simulink model "EZS4_template"  (R2017b)
settings: Solver=ode3  StartTime=0.0  StopTime=inf  RelTol=1e-3  EnableMultiTasking=on
libraries: arduinolib x13
settings Model: ExtModeTrigDuration=2  Creator=hartmann  LastModifiedBy=tanja
settings DataIOCC: LimitDataPoints=on  SaveFormat=Array
settings OptimizationCC: PassReuseOutputArgsThreshold=0  ExpressionDepthLimit=2147483647  MaxStackSize=64
settings DebuggingCC: UnderspecifiedInitializationDetection=Classic  MergeDetectMultiDrivingBlocksExec=none  ParameterTunabilityLossMsg=error  StateNameClashWarn=warning  SFUnexpectedBacktrackingDiag=warning  SFNoUnconditionalDefaultTransitionDiag=warning  SFExecutionAtInitializationDiag=none
settings HardwareCC: ProdBitPerInt=16  ProdBitPerPointer=16  ProdBitPerSizeT=16  ProdBitPerPtrDiffT=16  ProdLargestAtomicFloat=None  ProdWordSize=8  ProdHWDeviceType=Atmel->AVR  UseEmbeddedCoderFeatures=off  UseSimulinkCoderFeatures=off
settings ModelReferenceCC: PropagateSignalLabelsOutOfModel=off
settings SFSimCC: MATLABDynamicMemAlloc=off
settings RTWCC: SystemTargetFile=ert.tlc  HardwareBoard=Arduino Mega 2560  TLCOptions=-aInlineSetEventsForThisBaseRateFcn=TLC_FALSE -aSuppressMultiTaskScheduler=TLC_FALSE -aRateBasedStepFcn=1  TemplateMakefile=ert_default_tmf  GenerateReport=on  RTWVerbose=off  Toolchain=Arduino AVR  BuildConfiguration=Faster Runs  LaunchReport=on
settings CodeAppCC: ForceParamTrailComments=on  OperatorAnnotations=on
settings ERTTargetCC: ERTCustomFileBanners=off  SupportContinuousTime=on  SupportNonInlinedSFcns=on  RemoveResetFunc=off  SupportVariableSizeSignals=on  ModelStepFunctionPrototypeControlCompliant=off
settings ConfigComp: CovMetricSettings=dw  CovHtmlReporting=on  CovSaveCumulativeToWorkspaceVar=on  CovSaveSingleToWorkspaceVar=on  CovExternalEMLEnable=off  CovSFcnEnable=off

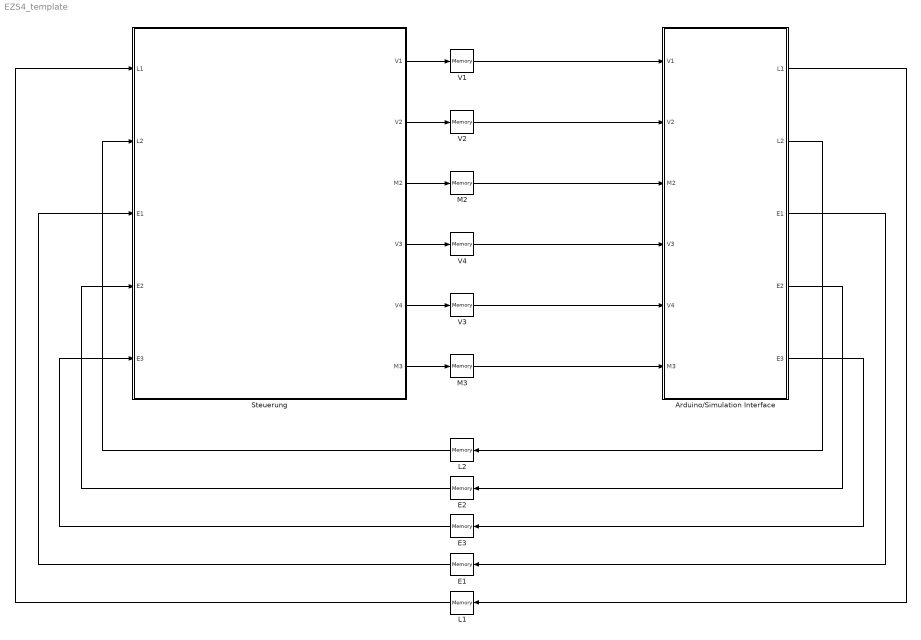
== system EZS4_template ==
  Arduino/Simulation Interface : Subsystem
  E1 : Memory
  E2 : Memory
  E3 : Memory
  L1 : Memory
  L2 : Memory
  M2 : Memory
  M3 : Memory
  Steuerung : Stateflow chart  TreatAsAtomicUnit=on
  V{1..4} (4 alike) : Memory
  wires:
  Steuerung/1(V1) -> V1/1
  Steuerung/2(V2) -> V2/1
  Steuerung/3(M2) -> M2/1
  Steuerung/6(M3) -> M3/1
  L1/1 -> Steuerung/1(L1)
  E1/1 -> Steuerung/3(E1)
  E3/1 -> Steuerung/5(E3)
  E2/1 -> Steuerung/4(E2)
  L2/1 -> Steuerung/2(L2)
  M3/1 -> Arduino/Simulation Interface/6("M3 ")
  V3/1 -> Arduino/Simulation Interface/5(V4)
  V4/1 -> Arduino/Simulation Interface/4(V3)
  M2/1 -> Arduino/Simulation Interface/3(M2)
  V2/1 -> Arduino/Simulation Interface/2(V2)
  V1/1 -> Arduino/Simulation Interface/1(V1)
  Arduino/Simulation Interface/1(L1) -> L1/1
  Arduino/Simulation Interface/2(L2) -> L2/1
  Arduino/Simulation Interface/3(E1) -> E1/1
  Arduino/Simulation Interface/4(E2) -> E2/1
  Arduino/Simulation Interface/5(E3) -> E3/1
  Steuerung/5(V4) -> V3/1
  Steuerung/4(V3) -> V4/1

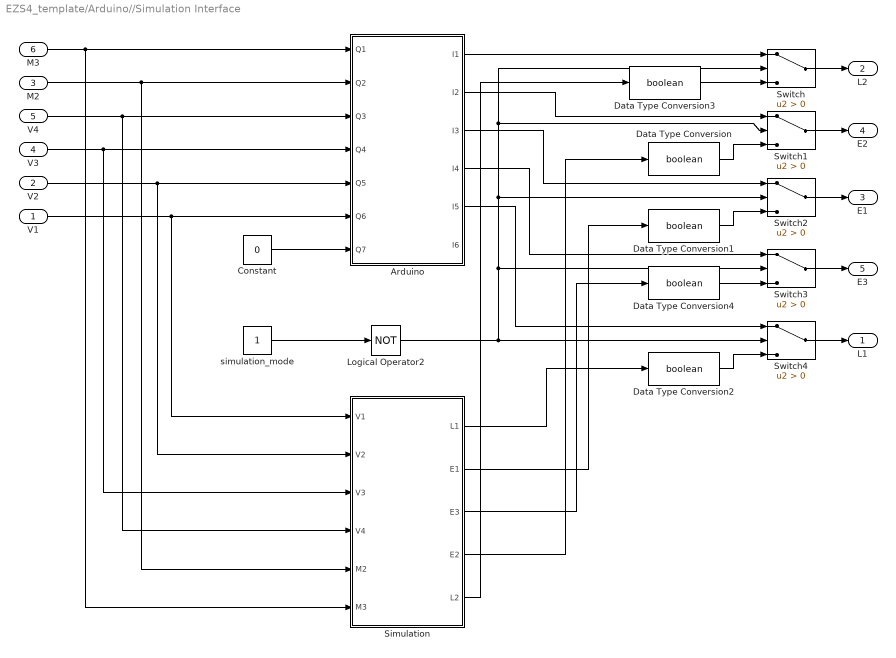
== system EZS4_template/Arduino//Simulation Interface ==
  V1 : Inport
  V2 : Inport  Port=2
  M2 : Inport  Port=3
  V3 : Inport  Port=4
  V4 : Inport  Port=5
  "M3 " : Inport  Port=6
  Arduino : Subsystem
  Constant : Constant  Value=0
  Data Type Conversion{,1..4} (5 alike) : DataTypeConversion  OutDataTypeStr=boolean
  Logical Operator2 : Logic  Operator=NOT  AllPortsSameDT=off  OutDataTypeStr=boolean
  Simulation : Stateflow chart  TreatAsAtomicUnit=on
  Switch{,1..4} (5 alike) : Switch  Criteria=u2 > Threshold
  simulation_mode : Constant
  L1 : Outport
  L2 : Outport  Port=2
  E1 : Outport  Port=3
  E2 : Outport  Port=4
  E3 : Outport  Port=5
  wires:
  Simulation/5(L2) -> Data Type Conversion3/1
  Switch/1 -> L2/1
  simulation_mode/1 -> Logical Operator2/1
  Arduino/1(I1) -> Switch/1
  Simulation/4(E2) -> Data Type Conversion/1
  Switch1/1 -> E2/1
  Arduino/2(I2) -> Switch1/1
  Data Type Conversion/1 -> Switch1/3
  Switch2/1 -> E1/1
  Simulation/2(E1) -> Data Type Conversion1/1
  Arduino/3(I3) -> Switch2/1
  Data Type Conversion1/1 -> Switch2/3
  Switch3/1 -> E3/1
  Simulation/3(E3) -> Data Type Conversion4/1
  Arduino/4(I4) -> Switch3/1
  Simulation/1(L1) -> Data Type Conversion2/1
  Switch4/1 -> L1/1
  Arduino/5(I5) -> Switch4/1
  Logical Operator2/1 -> Switch/2, Switch1/2, Switch2/2, Switch3/2, Switch4/2
  Constant/1 -> Arduino/7(Q7)
  V1/1 -> Simulation/1(V1), Arduino/6(Q6)
  V2/1 -> Simulation/2(V2), Arduino/5(Q5)
  M2/1 -> Simulation/5(M2), Arduino/2(Q2)
  V4/1 -> Arduino/3(Q3), Simulation/4(V4)
  V3/1 -> Arduino/4(Q4), Simulation/3(V3)
  "M3 "/1 -> Arduino/1(Q1), Simulation/6(M3)
  Data Type Conversion2/1 -> Switch4/3
  Data Type Conversion3/1 -> Switch/3
  Data Type Conversion4/1 -> Switch3/3

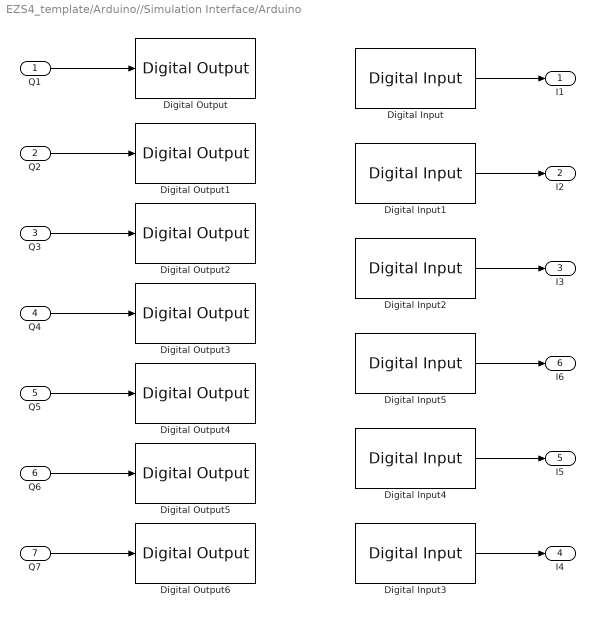
== system EZS4_template/Arduino//Simulation Interface/Arduino ==
  Q1 : Inport
  Q2 : Inport  Port=2
  Q3 : Inport  Port=3
  Q4 : Inport  Port=4
  Q5 : Inport  Port=5
  Q6 : Inport  Port=6
  Q7 : Inport  Port=7
  Digital Input : arduinolib/Digital Input  pinNumber=34  sampleTime=0.1  blockPlatform=arduino
      settings: SourceProductName=Simulink Support Package for Arduino Hardware
  Digital Input1 : arduinolib/Digital Input  pinNumber=36  sampleTime=0.1  blockPlatform=arduino
      settings: SourceProductName=Simulink Support Package for Arduino Hardware
  Digital Input2 : arduinolib/Digital Input  pinNumber=38  sampleTime=0.1  blockPlatform=arduino
      settings: SourceProductName=Simulink Support Package for Arduino Hardware
  Digital Input3 : arduinolib/Digital Input  pinNumber=44  sampleTime=0.1  blockPlatform=arduino
      settings: SourceProductName=Simulink Support Package for Arduino Hardware
  Digital Input4 : arduinolib/Digital Input  pinNumber=42  sampleTime=0.1  blockPlatform=arduino
      settings: SourceProductName=Simulink Support Package for Arduino Hardware
  Digital Input5 : arduinolib/Digital Input  pinNumber=40  sampleTime=0.1  blockPlatform=arduino
      settings: SourceProductName=Simulink Support Package for Arduino Hardware
  Digital Output : arduinolib/Digital Output  pinNumber=13  blockPlatform=arduino
  Digital Output1 : arduinolib/Digital Output  pinNumber=12  blockPlatform=arduino
  Digital Output2 : arduinolib/Digital Output  pinNumber=11  blockPlatform=arduino
  Digital Output3 : arduinolib/Digital Output  pinNumber=10  blockPlatform=arduino
  Digital Output4 : arduinolib/Digital Output  pinNumber=9  blockPlatform=arduino
  Digital Output5 : arduinolib/Digital Output  pinNumber=8  blockPlatform=arduino
  Digital Output6 : arduinolib/Digital Output  pinNumber=7  blockPlatform=arduino
  I1 : Outport
  I2 : Outport  Port=2
  I3 : Outport  Port=3
  I4 : Outport  Port=4
  I5 : Outport  Port=5
  I6 : Outport  Port=6
  wires:
  Q1/1 -> Digital Output/1
  Digital Input/1 -> I1/1
  Digital Input1/1 -> I2/1
  Digital Input2/1 -> I3/1
  Digital Input3/1 -> I4/1
  Digital Input4/1 -> I5/1
  Digital Input5/1 -> I6/1
  Q2/1 -> Digital Output1/1
  Q3/1 -> Digital Output2/1
  Q4/1 -> Digital Output3/1
  Q7/1 -> Digital Output6/1
  Q5/1 -> Digital Output4/1
  Q6/1 -> Digital Output5/1

== stateflow chart EZS4_template/Arduino//Simulation Interface/Simulation ==
  state default [parallel]
    du: L1=false;
    du: L2=false;
    du: E1=false;
    du: E2=false;
    du: E3=false;
    settings: executionOrder=1
  (default) -> default
  data: L1 output; V1 input; V2 input; V3 input; V4 input; M2 input; E1 output; E3 output; E2 output; L2 output; M3 input

== stateflow chart EZS4_template/Steuerung ==
  state default [parallel]
    du: V1=false;
    du: V2=false;
    du: V3=false;
    du: V4=false;
    du: M2=false;
    du: M3=false;
    settings: executionOrder=1
  data: L1 input; L2 input; E1 input; V1 output; V2 output; M2 output; V3 output; V4 output; M3 output; E2 input; E3 input
